simulink model "pneumatic_sampled_controller"  (R2025a)
settings: Solver=ode45  StartTime=0.0  StopTime=5  MaxStep=0.0005  RelTol=1e-8  AbsTol=1e-12
InitFcn:
  | addpath(fullfile(fileparts(get_param(bdroot,'FileName')),'matlab'));
model workspace (MAT data in the model file):
  controller_config = [35 1 2 0.7 0.6 200000 4]
  plant_parameters.R = 287.05
  plant_parameters.gamma = 1.4
  plant_parameters.temperature = 293.15
  plant_parameters.atmosphere = 101325
  plant_parameters.supply = 600000
  plant_parameters.bore = 0.02
  plant_parameters.rod = 0.008
  plant_parameters.stroke = 0.06
  plant_parameters.dead_volume = 5e-06
  plant_parameters.mass = 0.4
  plant_parameters.spring = 100
  plant_parameters.damping = 35
  plant_parameters.friction = 1
  plant_parameters.friction_velocity = 0.003
  plant_parameters.valve_area = 5e-07
  plant_parameters.discharge = 0.7
  plant_parameters.valve_tau = 0.025
  plant_parameters.leakage_area = 0
  plant_parameters.initial_position = 0.01
  plant_parameters.load = 2
  plant_parameters.kp = 100
  plant_parameters.ki = 30
  plant_parameters.kd = 5
  plant_parameters.stop_stiffness = 200000
  plant_parameters.stop_damping = 200
settings Model: Creator=dewar  LastModifiedBy=dewar

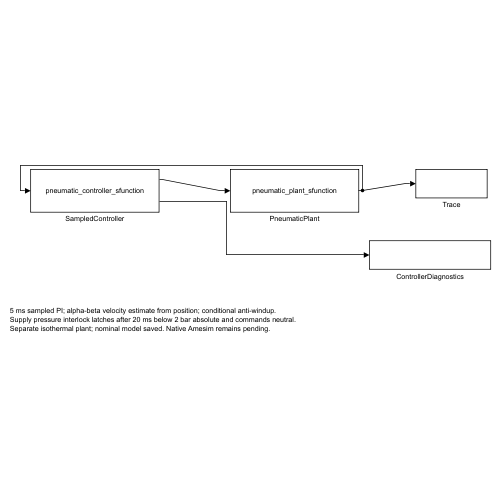
[thumbnail: Simulink's stored preview of the top-level diagram]
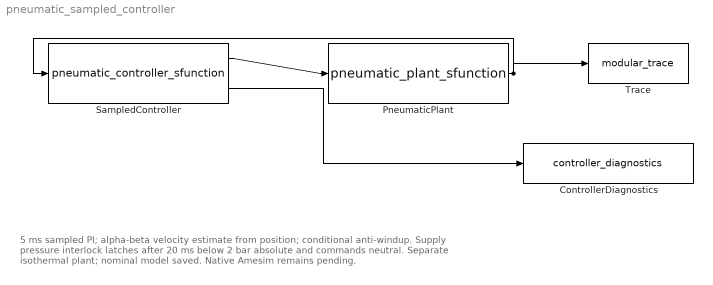
== system pneumatic_sampled_controller ==
  note: 5 ms sampled PI; alpha-beta velocity estimate from position; conditional anti-windup.
      | Supply pressure interlock latches after 20 ms below 2 bar absolute and commands neutral.
      | Separate isothermal plant; nominal model saved. Native Amesim remains pending.
  ControllerDiagnostics : ToWorkspace  VariableName=controller_diagnostics  SaveFormat=Structure With Time  SampleTime=-1
  PneumaticPlant : M-S-Function  FunctionName=pneumatic_plant_sfunction  Parameters=plant_parameters
  SampledController : M-S-Function  FunctionName=pneumatic_controller_sfunction  Parameters=controller_config
  Trace : ToWorkspace  VariableName=modular_trace  SaveFormat=Structure With Time  SampleTime=-1
  wires:
  SampledController/1 -> PneumaticPlant/1
  PneumaticPlant/1 -> SampledController/1, Trace/1
  SampledController/2 -> ControllerDiagnostics/1
